simulink subsystem "TractionEnergyConsumptionModel"  (R2024a)
settings: Solver=VariableStepAuto  StartTime=0.0  StopTime=10.0  RelTol=1e-3
values from neighbouring files (symbols this model uses):
  CdA = 6.62    [VehicleParameters.m]
  Cr = 0.00562    [VehicleParameters.m]
  m = 36000    [VehicleParameters.m]
  rho = 1.225    [VehicleParameters.m]
settings Model: Creator=44779  LastModifiedBy=44779

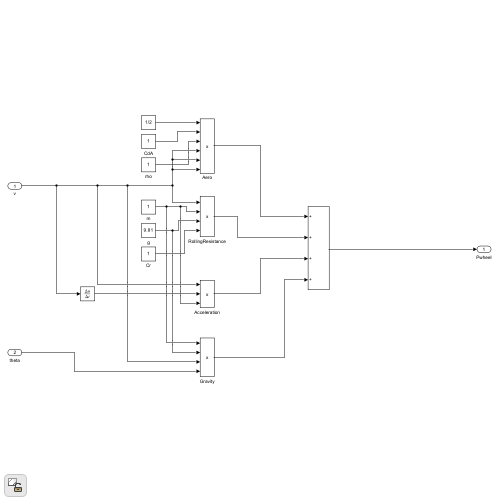
[thumbnail: Simulink's stored preview of the top-level diagram]
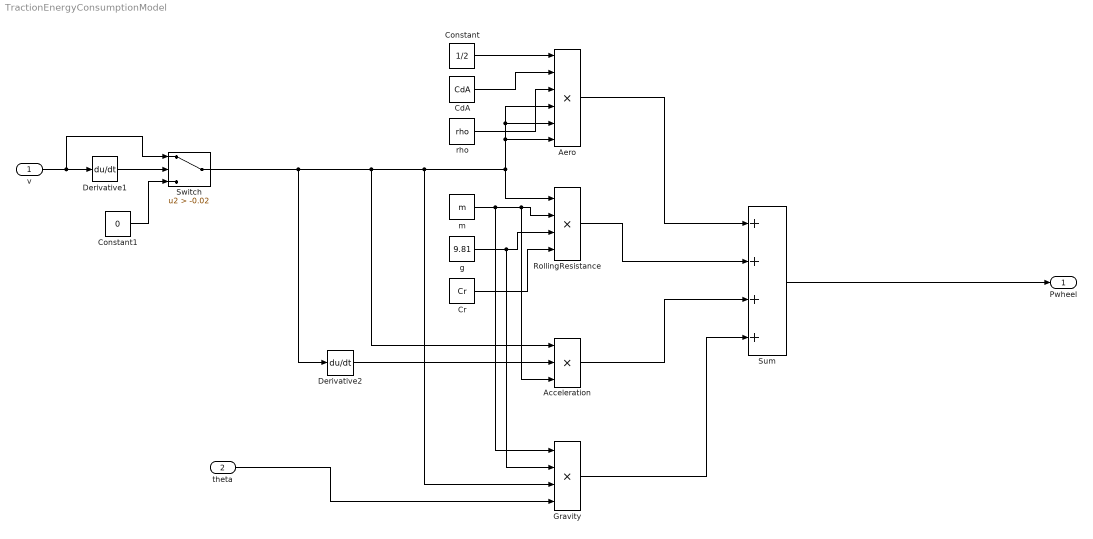
== system TractionEnergyConsumptionModel ==
  v : Inport
  theta : Inport  Port=2
  Acceleration : Product  Inputs=3
  Aero : Product  Inputs=6
  CdA : Constant  Value=CdA
  Constant : Constant  Value=1/2
  Constant1 : Constant  Value=0
  Cr : Constant  Value=Cr
  Derivative1 : Derivative
  Derivative2 : Derivative
  Gravity : Product  Inputs=4
  RollingResistance : Product  Inputs=4
  Sum : Sum  Inputs=++++
  Switch : Switch  Criteria=u2 > Threshold  Threshold=-0.02  SaturateOnIntegerOverflow=off  InputSameDT=off
  g : Constant  Value=9.81
  m : Constant  Value=m
  rho : Constant  Value=rho
  Pwheel : Outport
  wires:
  RollingResistance/1 -> Sum/2
  v/1 -> Derivative1/1, Switch/1
  m/1 -> RollingResistance/2, Acceleration/3, Gravity/1
  Gravity/1 -> Sum/4
  Cr/1 -> RollingResistance/4
  Aero/1 -> Sum/1
  Constant/1 -> Aero/1
  g/1 -> RollingResistance/3, Gravity/2
  theta/1 -> Gravity/4
  rho/1 -> Aero/3
  CdA/1 -> Aero/2
  Acceleration/1 -> Sum/3
  Sum/1 -> Pwheel/1
  Derivative1/1 -> Switch/2
  Switch/1 -> Aero/4, Aero/5, Aero/6, RollingResistance/1, Gravity/3, Acceleration/1, Derivative2/1
  Derivative2/1 -> Acceleration/2
  Constant1/1 -> Switch/3
